simulink library "Control_Unit_Simple"  (R2018b)
settings: Solver=VariableStepAuto  StartTime=0.0  StopTime=10.0  RelTol=1e-3
settings Model: Creator=Alexander Koch  LastModifiedBy=ga69qig
settings SFSimCC: SimUseLocalCustomCode=off
settings RTWCC: RTWUseLocalCustomCode=off
settings CodeAppCC: StateflowObjectComments=on

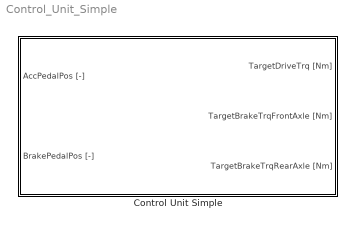
== system Control_Unit_Simple ==
  Control Unit Simple : Subsystem  mask(SB){Brake_Distribution_Front=0.7, MaxBrkTrq=1000, MaxMotorTrq=300, LocalSampleTime=-1}
      mask prompts: Brake_Distribution_Front "Brake Distribution Front"; MaxBrkTrq "Maximal Braking Torque"; MaxMotorTrq "Maximal Motor Torque"; LocalSampleTime "Local System Sample-Time [s]"
      mask help:
      | <Author> Alexander Koch, Benedikt Danquah based on Stefan Müller [1], Stephan Rohr [2]  </Author>
      | <Date> 03/04/2017 </Date>
      |
      | <Description>
      | Requires acceleration pedal position, braking pedal position, a brake distribution, the maximal possible braking torque and tha maximal motor torque and calculates a target drive system torque and a target braking torque for front and rear axle. Minimum drive torques is zero.
      | </Description>
      mask init:
      | GlobalSampleTime = CalcGlobalSampleTime(LocalSampleTime);
      mask Help:
      | <Parameters>
      | Brake distribution front [-]
      | 	<Min> 0 </Min>
      | 	<Max> 1 </Max>
      | Maximal braking torque [Nm]
      | Maximal motor torque [Nm]
      | Local System Sample-Time [s]
      | 	<Min> GlobalSampleTime </Min>
      | Global Sample-Time [s]
      | </Parameters>
      | 
      | <Inputs>
      | AccPedalPos [-]
      | 	<Min> 0 </Min>
      | 	<Max> 1 </Max>
      | BrakePedalPos [-]
      | 	<Min>0 </Min>
      | 	<Max> 1 </Max>
      | </Inputs>
      | 
      | <Outputs>
      | TargetDriveTrq [Nm]
      | 	<Min> 0 </Min>
      | TargetBrakeTrqFrontAxle [Nm]
      | 	<Max> 0 </Max>
      | TargetBrakeTrqRearAxle [Nm]
      | 	<Max> 0 </Max>
      | </Outputs>
      | <Sources>
      | [1] S. Mueller, S. Rohr, W. Schmid, and M. Lienkamp, “Analysing the Influence of Driver Behaviour and Tuning Measures on Battery Aging and Residual Value of Electric Vehicles,” in Proc. EVS30 Symposium, Stuttgart, 2017, pp. 1–12.
      | [2] S. Rohr, “Technisch-wirtschaftliche Analyse des Zweitnutzungs- potentials von Lithium-Ionen-Traktionsbatterien,” Dissertation, Institute of Automotive Technology, Technical University Munich, Munich, 2018.
      | </Sources>
      mask TypeOptions Brake_Distribution_Front: Brake_Distribution_Front/Value
      mask TypeOptions MaxBrkTrq: MaxBrakeTorque/Value
      mask TypeOptions MaxMotorTrq: MaxMotorTorque/Value
      mask TypeOptions LocalSampleTime: AccPedalPos [-]/SampleTime | BrakePedalPos [-]/SampleTime
      mask DialogControl Container3 Prompt: Documentation:
      mask DialogControl DescHelpVar Prompt: %<MaskHelp>
      mask DialogControl Container5 Prompt: Sample Time
      mask Display:
      | [picturexpos,pictureypos,picturewidth,pictureheight] = ...
      |     CalcBlockPicturePosition(gcb,1,0.01,0.1,80,120); % calculating picture position depending on Block size and minimum margin size
      | image('Control_Unit_Simple.svg',[picturexpos pictureypos picturewidth pictureheight]) % plot picture to block

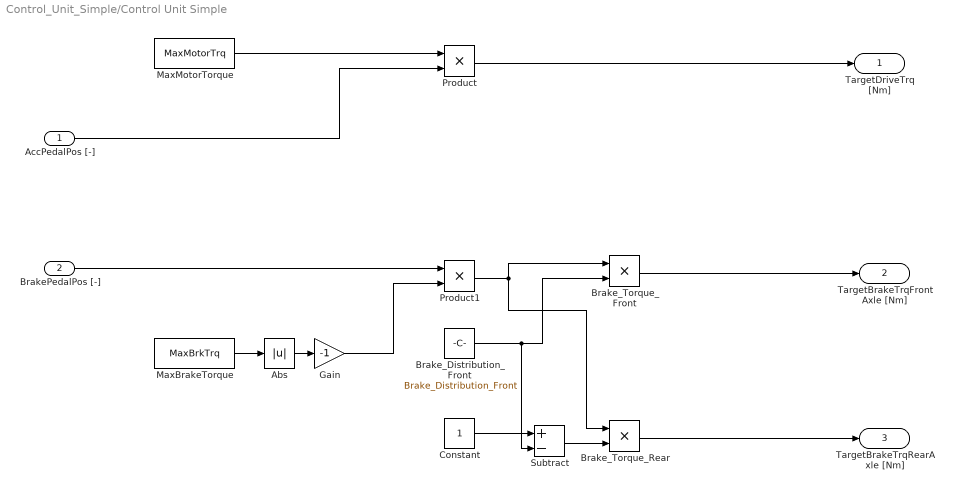
== system Control_Unit_Simple/Control Unit Simple ==
  AccPedalPos [-] : Inport  SampleTime=LocalSampleTime
  BrakePedalPos [-] : Inport  Port=2  SampleTime=LocalSampleTime
  Abs : Abs
  Brake_Distribution_Front : Constant  Value=Brake_Distribution_Front
  Brake_Torque_Front : Product
  Brake_Torque_Rear : Product
  Constant : Constant
  Gain : Gain  Gain=-1
  MaxBrakeTorque : Constant  Value=MaxBrkTrq
  MaxMotorTorque : Constant  Value=MaxMotorTrq
  Product : Product
  Product1 : Product
  Subtract : Sum  Inputs=+-
  "TargetDriveTrq [Nm] " : Outport  SampleTime=GlobalSampleTime
  TargetBrakeTrqFrontAxle [Nm] : Outport  Port=2  SampleTime=GlobalSampleTime
  TargetBrakeTrqRearAxle [Nm] : Outport  Port=3  SampleTime=GlobalSampleTime
  wires:
  Product/1 -> "TargetDriveTrq [Nm] "/1
  BrakePedalPos [-]/1 -> Product1/1
  Brake_Torque_Front/1 -> TargetBrakeTrqFrontAxle [Nm]/1
  MaxMotorTorque/1 -> Product/1
  Subtract/1 -> Brake_Torque_Rear/2
  Constant/1 -> Subtract/1
  AccPedalPos [-]/1 -> Product/2
  Brake_Torque_Rear/1 -> TargetBrakeTrqRearAxle [Nm]/1
  MaxBrakeTorque/1 -> Abs/1
  Brake_Distribution_Front/1 -> Subtract/2, Brake_Torque_Front/2
  Product1/1 -> Brake_Torque_Rear/1, Brake_Torque_Front/1
  Abs/1 -> Gain/1
  Gain/1 -> Product1/2
